simulink model "Fuzzy_PD_Controller_new"  (R2014b)
settings: Solver=ode45  StartTime=0.0  StopTime=20  RelTol=1e-3
undefined symbols (not defined in the file or in its folder): sigbuilder_block
libraries: simulink x1, fuzblock x1
settings Model: ExtModeTrigDuration=100  Creator=Asus  LastModifiedBy=Asus
settings SolverCC: ZeroCrossControl=DisableAll
settings DataIOCC: SaveFinalState=on  SaveFormat=StructureWithTime  SaveOutput=off  SaveState=on  StateSaveName=tmp_raccel_xout  SignalLoggingName=tmp_raccel_logsout
settings OptimizationCC: EfficientMapNaN2IntZero=off
settings DebuggingCC: SolverPrmCheckMsg=none
settings HardwareCC: TargetLongLongMode=on  TargetIntDivRoundTo=Zero  TargetEndianess=LittleEndian  TargetHWDeviceType=MATLAB Host  ProdEqTarget=off
settings RTWCC: SystemTargetFile=raccel.tlc  TemplateMakefile=raccel_default_tmf  RTWVerbose=off  ProcessScript=raccel_make_rtw_hook  RTWUseSimCustomCode=on
settings CodeAppCC: GenerateComments=off  MaxIdLength=128  MangleLength=10  SimulinkBlockComments=off
settings RaccelTargetCC: ERTMultiwordTypeDef=System defined  ERTMultiwordLength=256  GeneratePreprocessorConditionals=Disable all  ERTFirstTimeCompliant=off  MultiInstanceERTCode=off  EnableShiftOperators=on  ExtModeMexArgs='', 0, 21850  ENABLE_SLEXEC_SSBRIDGE=0  RTWCAPIParams=off

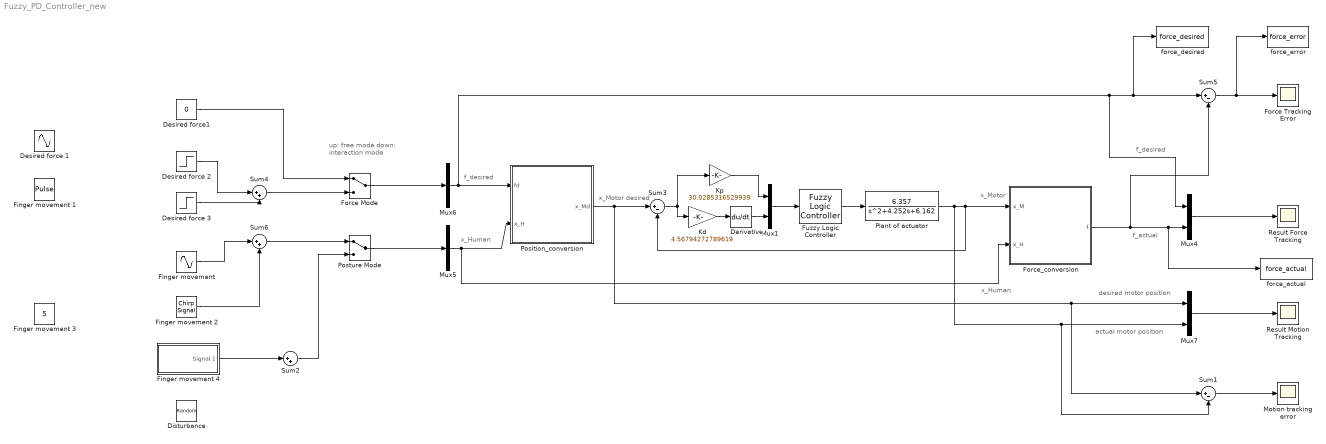
== system Fuzzy_PD_Controller_new ==
  note: x_Motor
  note: x_Motor desired
  note: x_Human
  note: actual motor position
  note: desired motor position
  note: f_desired
  note: f_actual
  note: x_Human
  note: f_desired
  note: up: free mode
      | down: interaction mode
  Derivative : Derivative
  Desired force 1 : Sin  Samples=20  SampleTime=0
  Desired force 2 : Step  Time=3  After=5  SampleTime=0
  Desired force 3 : Step  Time=6  After=-5  SampleTime=0
  Desired force1 : Constant  Value=0
  Disturbance : RandomNumber  Variance=0.2  SampleTime=0.1
  Finger movement 1 : DiscretePulseGenerator  PulseType=Time based  Period=5  PulseWidth=50
  Finger movement : Sin  Bias=8  Frequency=2  Samples=20  SampleTime=0
  Finger movement 2 : simulink/Sources/Chirp Signal  f1=0  T=20  f2=1
  Finger movement 3 : Constant  Value=5
  Finger movement 4 : Subsystem  Tag=STV Subsys  LoadFcn=sigbuilder_block('load');  StartFcn=sigbuilder_block('start');  StopFcn=sigbuilder_block('stop');  ClipboardFcn=sigbuilder_block('clipboard');  mask(Sigbuilder block){}
      mask help: Simulink:masks:SigbuilderBlock_MD
      mask init:
      | if ~strcmp(get_param(bdroot(gcbh),'SimulationStatus'),'stopped') tuvar = sigbuilder_block('maskInit'); end
      settings: CopyFcn=sigbuilder_block('copy');  DeleteFcn=sigbuilder_block('delete');  ModelCloseFcn=sigbuilder_block('modelClose');  PreSaveFcn=sigbuilder_block('preSave');  PauseFcn=sigbuilder_block('pause');  ContinueFcn=sigbuilder_block('continue');  NameChangeFcn=sigbuilder_block('namechange');  OpenFcn=sigbuilder_block('open',[437.6 199.2 550.4 400 ]);  CloseFcn=sigbuilder_block('close');
      mask Display: plot(0, 0, 100, 100,[2, 2, 32, 32, 2], [68, 8, 8, 68, 68],[32, 2], [38, 38], [32, 19, 2],[53, 60, 44], [32, 17, 17, 2],[16, 16, 31, 31]);txt = getActiveGroup(gcbh);text(2, 100, txt,'verticalAlignment', 'top');
  Force Mode : ManualSwitch
  Force Tracking Error : Scope
      settings: ShowLegends=on  SaveName=ScopeData5
  Force_conversion : MATLAB Function  TreatAsAtomicUnit=on
  Fuzzy Logic Controller : fuzblock/Fuzzy Logic  Controller  fis=['Fuzzy_controller_new.fis']
  Kd : Gain  Gain=4.56794272789619
  Kp : Gain  Gain=30.0285316529939
  Motion tracking error : Scope
      settings: ShowLegends=on
  Mux1 : Mux  Inputs=2
  Mux4 : Mux  Inputs=2
  Mux5 : Mux  Inputs=1
  Mux6 : Mux  Inputs=1
  Mux7 : Mux  Inputs=2
  Plant of actuator : TransferFcn  Numerator=[6.357]  Denominator=[1 4.252 6.162]
  Position_conversion : MATLAB Function  TreatAsAtomicUnit=on
  Posture Mode : ManualSwitch
  Result Force Tracking : Scope
      settings: ShowLegends=on  SaveName=ScopeData4
  Result Motion Tracking : Scope
      settings: ShowLegends=on  SaveName=ScopeData3
  Sum1 : Sum  Inputs=|+-
  Sum2 : Sum  Inputs=|++
  Sum3 : Sum  Inputs=|+-
  Sum4 : Sum  Inputs=|++
  Sum5 : Sum  Inputs=|+-
  Sum6 : Sum  Inputs=|++
  "force_actual " : ToWorkspace  VariableName=force_actual  SampleTime=-1
      settings: Save2DSignal=2-D array (concatenate along first dimension)
  force_desired : ToWorkspace  VariableName=force_desired  SampleTime=-1
      settings: Save2DSignal=2-D array (concatenate along first dimension)
  force_error : ToWorkspace  VariableName=force_error  SampleTime=-1
      settings: Save2DSignal=2-D array (concatenate along first dimension)
  wires:
  Position_conversion/1(x_Md) -> Sum1/1, Mux7/1, Sum3/1
  Force_conversion/1(f) -> Sum5/2, "force_actual "/1, Mux4/2
  Mux5/1 -> Force_conversion/2(x_H), Position_conversion/2(x_H)
  Mux6/1 -> Mux4/1, force_desired/1, Sum5/1, Position_conversion/1(fd)
  Mux7/1 -> Result Motion Tracking/1
  Sum5/1 -> force_error/1, Force Tracking Error/1
  Mux4/1 -> Result Force Tracking/1
  Sum1/1 -> Motion tracking error/1
  Derivative/1 -> Mux1/2
  Mux1/1 -> Fuzzy Logic Controller/1
  Fuzzy Logic Controller/1 -> Plant of actuator/1
  Kd/1 -> Derivative/1
  Sum3/1 -> Kd/1, Kp/1
  Kp/1 -> Mux1/1
  Desired force 3/1 -> Sum4/2
  Desired force 2/1 -> Sum4/1
  Sum4/1 -> Force Mode/2
  Force Mode/1 -> Mux6/1
  Posture Mode/1 -> Mux5/1
  Desired force1/1 -> Force Mode/1
  Finger movement/1 -> Sum6/1
  Sum6/1 -> Posture Mode/1
  Finger movement 2/1 -> Sum6/2
  Finger movement 4/1(Signal 1) -> Sum2/1
  Sum2/1 -> Posture Mode/2
  Plant of actuator/1 -> Sum1/2, Mux7/2, Sum3/2, Force_conversion/1(x_M)

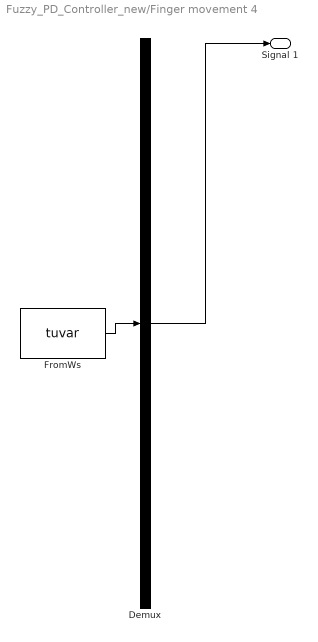
== system Fuzzy_PD_Controller_new/Finger movement 4 ==
  Demux : Demux  Tag=STV Demux  Outputs=1
  FromWs : FromWorkspace  Tag=STV FromWs  VariableName=tuvar  SampleTime=0
      SigBuilderData=|
      | common.afterFinalStr = 'Extrapolate'
      | common.sampleTime = 0
      | dataSet.timeRange = [0 10]
      | dataSet.name = 'Group 1'
      | sbobj.Groups.Name = 'Group 1'
      | sbobj.Groups.Signals.Name = 'Signal 1'
      | sbobj.Groups.Signals.XData = [0 3 6 10]
      | sbobj.Groups.Signals.YData = [8 13 13 8]
  Signal 1 : Outport  Tag=STV Outport
  wires:
  Demux/1 -> Signal 1/1
  FromWs/1 -> Demux/1

== matlab function Fuzzy_PD_Controller_new/Force_conversion ==
  data: x_M input; f output; x_H input
function f = force_conver(x_M,x_H)
%#codegen
    k = 0.434;
    L0 = 8;
    f = k*(x_H - x_M - L0);
end

== matlab function Fuzzy_PD_Controller_new/Position_conversion ==
  data: fd input; x_Md output; x_H input
function x_Md = pos_conver(fd,x_H)
%#codegen
    k = 0.434; %N/mm
    L0 = 8;    %mm
    x_Md = x_H - (fd/k) - L0;
end
